simulink model "gm_CustArch_vnl"  (R2020a)
settings: Solver=FixedStepDiscrete  StartTime=0.0  StopTime=7e4  RelTol=1e-3
libraries: simulink x176, hdlsllib x104, hdlmdlgenlib x2, dsparch4 x1
(part 4 of 4)

== system gm_CustArch_vnl/cust_architecture_vnl/output_interpret/Interpret_to_RAM_output/get enabled timings /Subsystem ==
  note: this is the ugliest thing ever--- but it works.. so far so good
  "counter " : Inport
  data_stream_en : Inport  Port=2
  Bit Rotate : hdlsllib/Logic and Bit Operations/Bit Rotate  mode=Rotate Right  N=1
      settings: SourceProductBaseCode=SL
  Bit Rotate1 : hdlsllib/Logic and Bit Operations/Bit Rotate  mode=Rotate Right  N=2
      settings: SourceProductBaseCode=SL
  Bit Rotate2 : hdlsllib/Logic and Bit Operations/Bit Rotate  mode=Rotate Right  N=3
      settings: SourceProductBaseCode=SL
  Bit Rotate3 : hdlsllib/Logic and Bit Operations/Bit Rotate  mode=Rotate Right  N=4
      settings: SourceProductBaseCode=SL
  Bit Rotate4 : hdlsllib/Logic and Bit Operations/Bit Rotate  mode=Rotate Right  N=5
      settings: SourceProductBaseCode=SL
  Bit Rotate5 : hdlsllib/Logic and Bit Operations/Bit Rotate  mode=Rotate Right  N=6
      settings: SourceProductBaseCode=SL
  Bit Rotate6 : hdlsllib/Logic and Bit Operations/Bit Rotate  mode=Rotate Right  N=7
      settings: SourceProductBaseCode=SL
  Bit Slice : hdlsllib/Logic and Bit Operations/Bit Slice  lidx=0  ridx=0
      settings: SourceProductBaseCode=SL
  Compare To Constant : simulink/Logic and Bit Operations/Compare To Constant  relop===  const=0  OutDataTypeStr=boolean
  Compare To Constant1 : simulink/Logic and Bit Operations/Compare To Constant  relop===  const=1  OutDataTypeStr=boolean
  Compare To Constant2 : simulink/Logic and Bit Operations/Compare To Constant  relop===  const=2  OutDataTypeStr=boolean
  Compare To Constant3 : simulink/Logic and Bit Operations/Compare To Constant  relop===  const=3  OutDataTypeStr=boolean
  Compare To Constant4 : simulink/Logic and Bit Operations/Compare To Constant  relop===  const=4  OutDataTypeStr=boolean
  Compare To Constant5 : simulink/Logic and Bit Operations/Compare To Constant  relop===  const=5  OutDataTypeStr=boolean
  Compare To Constant6 : simulink/Logic and Bit Operations/Compare To Constant  relop===  const=6  OutDataTypeStr=boolean
  Compare To Constant7 : simulink/Logic and Bit Operations/Compare To Constant  relop===  const=7  OutDataTypeStr=boolean
  Constant : Constant  Value=0  OutDataTypeStr=uint8  SampleTime=-1
  Switch{,1..7} (8 alike) : Switch  Criteria=u2 > Threshold
  source_device_en : Outport  VectorParamsAs1DForOutWhenUnconnected=off
  source_device : Outport  Port=2  VectorParamsAs1DForOutWhenUnconnected=off
  wires:
  Bit Slice/1 -> source_device_en/1
  Switch/1 -> Bit Slice/1
  data_stream_en/1 -> Bit Rotate6/1, Bit Rotate5/1, Bit Rotate4/1, Bit Rotate3/1, Bit Rotate2/1, Bit Rotate1/1, Bit Rotate/1, Switch/1
  Switch2/1 -> Switch1/3
  Constant/1 -> Switch7/3
  Bit Rotate6/1 -> Switch7/1
  Switch7/1 -> Switch6/3
  Compare To Constant7/1 -> Switch7/2
  Bit Rotate5/1 -> Switch6/1
  Switch6/1 -> Switch5/3
  Compare To Constant6/1 -> Switch6/2
  Switch5/1 -> Switch4/3
  Bit Rotate4/1 -> Switch5/1
  Compare To Constant5/1 -> Switch5/2
  Bit Rotate3/1 -> Switch4/1
  Switch4/1 -> Switch3/3
  Compare To Constant4/1 -> Switch4/2
  Bit Rotate2/1 -> Switch3/1
  Switch3/1 -> Switch2/3
  Compare To Constant3/1 -> Switch3/2
  Bit Rotate1/1 -> Switch2/1
  Compare To Constant2/1 -> Switch2/2
  Switch1/1 -> Switch/3
  "counter "/1 -> source_device/1, Compare To Constant/1, Compare To Constant1/1, Compare To Constant2/1, Compare To Constant3/1, Compare To Constant4/1, Compare To Constant5/1, Compare To Constant6/1, Compare To Constant7/1
  Bit Rotate/1 -> Switch1/1
  Compare To Constant1/1 -> Switch1/2
  Compare To Constant/1 -> Switch/2

== system gm_CustArch_vnl/cust_architecture_vnl/output_interpret/Interpret_to_RAM_output/get enabled timings /Triggered Subsystem ==
  In1 : Inport
  Trigger : TriggerPort  VariantControl=Variant
  Bit Rotate : hdlsllib/Logic and Bit Operations/Bit Rotate  mode=Rotate Right  N=1
      settings: SourceProductBaseCode=SL
  Out1 : Outport  InitialOutput=0  VectorParamsAs1DForOutWhenUnconnected=off
  wires:
  Bit Rotate/1 -> Out1/1
  In1/1 -> Bit Rotate/1

== system gm_CustArch_vnl/cust_architecture/input_interpret_store_retrieve/Interpret_to_RAM_input/interpret data/get_sources/Subsystem ==
  source_device : Inport  OutDataTypeStr=uint8  PortDimensions=1  SampleTime=1
  dev_output : Inport  Port=2  OutDataTypeStr=uint8  PortDimensions=1  SampleTime=1
  Enable : EnablePort  OutDataTypeStr=boolean
  Bit Concat : hdlsllib/Logic and Bit Operations/Bit Concat  numInputs=2
  Bit Slice : hdlsllib/Logic and Bit Operations/Bit Slice  lidx=double(4)  ridx=double(0)
      settings: SourceProductBaseCode=SL
  Bit Slice1 : hdlsllib/Logic and Bit Operations/Bit Slice  lidx=double(2)  ridx=double(0)
      settings: SourceProductBaseCode=SL
  source_channel_0_159 : Outport  InitialOutput=0  VectorParamsAs1DForOutWhenUnconnected=off
  wires:
  Bit Slice1/1 -> Bit Concat/2
  Bit Slice/1 -> Bit Concat/1
  Bit Concat/1 -> source_channel_0_159/1
  dev_output/1 -> Bit Slice/1
  source_device/1 -> Bit Slice1/1

== system gm_CustArch_vnl/cust_architecture/input_interpret_store_retrieve/Interpret_to_RAM_input/interpret data/get_sources/Triggered Subsystem ==
  In1 : Inport  OutDataTypeStr=uint8  PortDimensions=1  SampleTime=1
  Enable : EnablePort  OutDataTypeStr=boolean
  Out1 : Outport  InitialOutput=0  VectorParamsAs1DForOutWhenUnconnected=off
  wires:
  In1/1 -> Out1/1

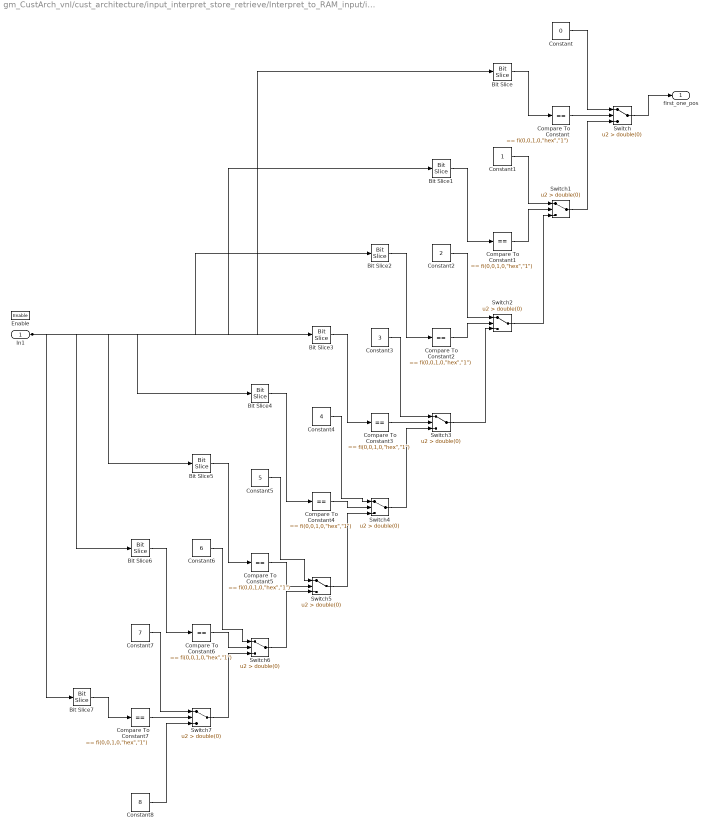
== system gm_CustArch_vnl/cust_architecture/input_interpret_store_retrieve/Interpret_to_RAM_input/interpret data/get_sources/find_first_one_pos ==
  In1 : Inport  OutDataTypeStr=uint8  PortDimensions=1  SampleTime=1
  Enable : EnablePort  OutDataTypeStr=boolean
  Bit Slice : hdlsllib/Logic and Bit Operations/Bit Slice  lidx=double(0)  ridx=double(0)
      settings: SourceProductBaseCode=SL
  Bit Slice1 : hdlsllib/Logic and Bit Operations/Bit Slice  lidx=double(1)  ridx=double(1)
      settings: SourceProductBaseCode=SL
  Bit Slice2 : hdlsllib/Logic and Bit Operations/Bit Slice  lidx=double(2)  ridx=double(2)
      settings: SourceProductBaseCode=SL
  Bit Slice3 : hdlsllib/Logic and Bit Operations/Bit Slice  lidx=double(3)  ridx=double(3)
      settings: SourceProductBaseCode=SL
  Bit Slice4 : hdlsllib/Logic and Bit Operations/Bit Slice  lidx=double(4)  ridx=double(4)
      settings: SourceProductBaseCode=SL
  Bit Slice5 : hdlsllib/Logic and Bit Operations/Bit Slice  lidx=double(5)  ridx=double(5)
      settings: SourceProductBaseCode=SL
  Bit Slice6 : hdlsllib/Logic and Bit Operations/Bit Slice  lidx=double(6)  ridx=double(6)
      settings: SourceProductBaseCode=SL
  Bit Slice7 : hdlsllib/Logic and Bit Operations/Bit Slice  lidx=double(7)  ridx=double(7)
      settings: SourceProductBaseCode=SL
  Compare To Constant{,1..7} (8 alike) : simulink/Logic and Bit Operations/Compare To Constant  relop===  const="fi(0,0,1,0,\"hex\",\"1\")"  OutDataTypeStr=boolean
  Constant : Constant  Value=0  OutDataTypeStr=uint8  SampleTime=1
  Constant1 : Constant  OutDataTypeStr=uint8  SampleTime=1
  Constant2 : Constant  Value=2  OutDataTypeStr=uint8  SampleTime=1
  Constant3 : Constant  Value=3  OutDataTypeStr=uint8  SampleTime=1
  Constant4 : Constant  Value=4  OutDataTypeStr=uint8  SampleTime=1
  Constant5 : Constant  Value=5  OutDataTypeStr=uint8  SampleTime=1
  Constant6 : Constant  Value=6  OutDataTypeStr=uint8  SampleTime=1
  Constant7 : Constant  Value=7  OutDataTypeStr=uint8  SampleTime=1
  Constant8 : Constant  Value=8  OutDataTypeStr=uint8  SampleTime=1
  Switch{,1..7} (8 alike) : Switch  Criteria=u2 > Threshold  Threshold=double(0)  OutDataTypeStr=uint8  SampleTime=1
  first_one_pos : Outport  InitialOutput=0  VectorParamsAs1DForOutWhenUnconnected=off
  wires:
  Switch7/1 -> Switch6/3
  Switch6/1 -> Switch5/3
  Switch5/1 -> Switch4/3
  Switch4/1 -> Switch3/3
  Switch3/1 -> Switch2/3
  Switch2/1 -> Switch1/3
  Switch1/1 -> Switch/3
  Switch/1 -> first_one_pos/1
  Constant8/1 -> Switch7/3
  Constant7/1 -> Switch7/1
  Constant6/1 -> Switch6/1
  Constant5/1 -> Switch5/1
  Constant4/1 -> Switch4/1
  Constant3/1 -> Switch3/1
  Constant2/1 -> Switch2/1
  Constant1/1 -> Switch1/1
  Constant/1 -> Switch/1
  Compare To Constant7/1 -> Switch7/2
  Compare To Constant6/1 -> Switch6/2
  Compare To Constant5/1 -> Switch5/2
  Compare To Constant4/1 -> Switch4/2
  Compare To Constant3/1 -> Switch3/2
  Compare To Constant2/1 -> Switch2/2
  Compare To Constant1/1 -> Switch1/2
  Compare To Constant/1 -> Switch/2
  Bit Slice7/1 -> Compare To Constant7/1
  Bit Slice6/1 -> Compare To Constant6/1
  Bit Slice5/1 -> Compare To Constant5/1
  Bit Slice4/1 -> Compare To Constant4/1
  Bit Slice3/1 -> Compare To Constant3/1
  Bit Slice2/1 -> Compare To Constant2/1
  Bit Slice1/1 -> Compare To Constant1/1
  Bit Slice/1 -> Compare To Constant/1
  In1/1 -> Bit Slice/1, Bit Slice1/1, Bit Slice2/1, Bit Slice3/1, Bit Slice4/1, Bit Slice5/1, Bit Slice6/1, Bit Slice7/1

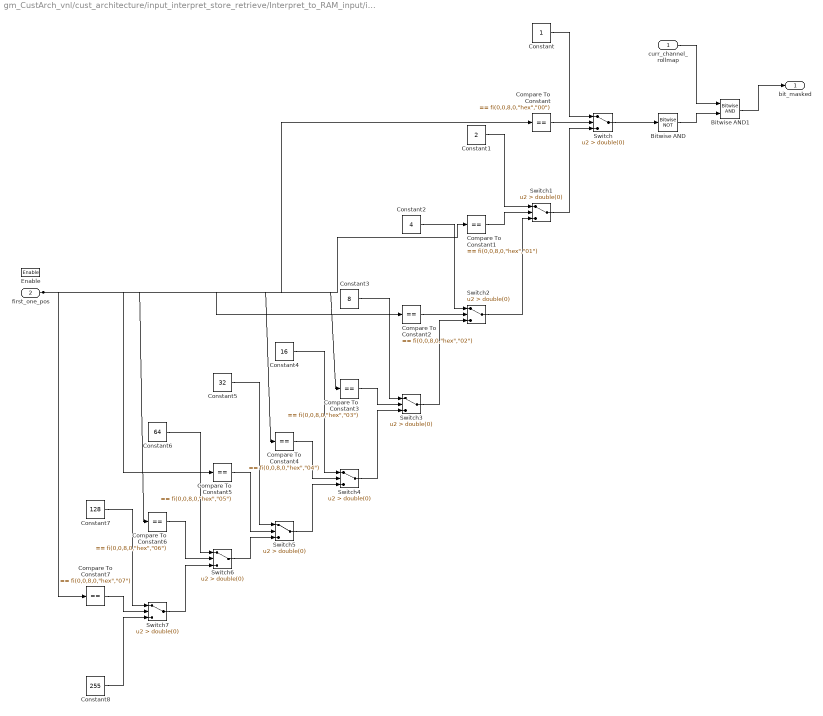
== system gm_CustArch_vnl/cust_architecture/input_interpret_store_retrieve/Interpret_to_RAM_input/interpret data/get_sources/position_to_bitmask ==
  curr_channel_rollmap : Inport  OutDataTypeStr=uint8  PortDimensions=1  SampleTime=1
  first_one_pos : Inport  Port=2  OutDataTypeStr=uint8  PortDimensions=1  SampleTime=1
  Enable : EnablePort  OutDataTypeStr=boolean
  Bitwise AND : simulink/Logic and Bit Operations/Bitwise Operator  logicop=NOT  UseBitMask=off  BitMask=double(0)  BitMaskRealWorld=Real World Value
  Bitwise AND1 : simulink/Logic and Bit Operations/Bitwise Operator  logicop=AND  UseBitMask=off  NumInputPorts=2  BitMask=double(0)  BitMaskRealWorld=Real World Value
  Compare To Constant : simulink/Logic and Bit Operations/Compare To Constant  relop===  const="fi(0,0,8,0,\"hex\",\"00\")"  OutDataTypeStr=boolean
  Compare To Constant1 : simulink/Logic and Bit Operations/Compare To Constant  relop===  const="fi(0,0,8,0,\"hex\",\"01\")"  OutDataTypeStr=boolean
  Compare To Constant2 : simulink/Logic and Bit Operations/Compare To Constant  relop===  const="fi(0,0,8,0,\"hex\",\"02\")"  OutDataTypeStr=boolean
  Compare To Constant3 : simulink/Logic and Bit Operations/Compare To Constant  relop===  const="fi(0,0,8,0,\"hex\",\"03\")"  OutDataTypeStr=boolean
  Compare To Constant4 : simulink/Logic and Bit Operations/Compare To Constant  relop===  const="fi(0,0,8,0,\"hex\",\"04\")"  OutDataTypeStr=boolean
  Compare To Constant5 : simulink/Logic and Bit Operations/Compare To Constant  relop===  const="fi(0,0,8,0,\"hex\",\"05\")"  OutDataTypeStr=boolean
  Compare To Constant6 : simulink/Logic and Bit Operations/Compare To Constant  relop===  const="fi(0,0,8,0,\"hex\",\"06\")"  OutDataTypeStr=boolean
  Compare To Constant7 : simulink/Logic and Bit Operations/Compare To Constant  relop===  const="fi(0,0,8,0,\"hex\",\"07\")"  OutDataTypeStr=boolean
  Constant : Constant  OutDataTypeStr=uint8  SampleTime=1
  Constant1 : Constant  Value=2  OutDataTypeStr=uint8  SampleTime=1
  Constant2 : Constant  Value=4  OutDataTypeStr=uint8  SampleTime=1
  Constant3 : Constant  Value=8  OutDataTypeStr=uint8  SampleTime=1
  Constant4 : Constant  Value=16  OutDataTypeStr=uint8  SampleTime=1
  Constant5 : Constant  Value=32  OutDataTypeStr=uint8  SampleTime=1
  Constant6 : Constant  Value=64  OutDataTypeStr=uint8  SampleTime=1
  Constant7 : Constant  Value=128  OutDataTypeStr=uint8  SampleTime=1
  Constant8 : Constant  Value=255  OutDataTypeStr=uint8  SampleTime=1
  Switch{,1..7} (8 alike) : Switch  Criteria=u2 > Threshold  Threshold=double(0)  OutDataTypeStr=uint8  SampleTime=1
  bit_masked : Outport  InitialOutput=0  VectorParamsAs1DForOutWhenUnconnected=off
  wires:
  Switch7/1 -> Switch6/3
  Switch6/1 -> Switch5/3
  Switch5/1 -> Switch4/3
  Switch4/1 -> Switch3/3
  Switch3/1 -> Switch2/3
  Switch2/1 -> Switch1/3
  Switch1/1 -> Switch/3
  Switch/1 -> Bitwise AND/1
  Constant8/1 -> Switch7/3
  Constant7/1 -> Switch7/1
  Constant6/1 -> Switch6/1
  Constant5/1 -> Switch5/1
  Constant4/1 -> Switch4/1
  Constant3/1 -> Switch3/1
  Constant2/1 -> Switch2/1
  Constant1/1 -> Switch1/1
  Constant/1 -> Switch/1
  Compare To Constant7/1 -> Switch7/2
  Compare To Constant6/1 -> Switch6/2
  Compare To Constant5/1 -> Switch5/2
  Compare To Constant4/1 -> Switch4/2
  Compare To Constant3/1 -> Switch3/2
  Compare To Constant2/1 -> Switch2/2
  Compare To Constant1/1 -> Switch1/2
  Compare To Constant/1 -> Switch/2
  Bitwise AND1/1 -> bit_masked/1
  Bitwise AND/1 -> Bitwise AND1/2
  first_one_pos/1 -> Compare To Constant/1, Compare To Constant1/1, Compare To Constant2/1, Compare To Constant3/1, Compare To Constant4/1, Compare To Constant5/1, Compare To Constant6/1, Compare To Constant7/1
  curr_channel_rollmap/1 -> Bitwise AND1/1

== system gm_CustArch_vnl/cust_architecture/process_and_retrieve/80-120Hz IIR/controlss_temp/Filter/delay_process_section10_tap0 ==
  in0 : Inport  OutDataTypeStr=fixdt(1, 16, 15)  SampleTime=1
  Trigger_emulated : EnablePort  OutDataTypeStr=boolean
  delay_process_section10_tap0 : Delay  DelayLength=double(1)
  out0 : Outport  OutDataTypeStr=fixdt(1, 16, 15)  InitialOutput=0
  wires:
  in0/1 -> delay_process_section10_tap0/1
  delay_process_section10_tap0/1 -> out0/1

== system gm_CustArch_vnl/cust_architecture/process_and_retrieve/80-120Hz IIR/controlss_temp/Filter/delay_process_section10_tap1 ==
  in0 : Inport  OutDataTypeStr=fixdt(1, 16, 15)  SampleTime=1
  Trigger_emulated : EnablePort  OutDataTypeStr=boolean
  delay_process_section10_tap1 : Delay  DelayLength=double(1)
  out0 : Outport  OutDataTypeStr=fixdt(1, 16, 15)  InitialOutput=0
  wires:
  in0/1 -> delay_process_section10_tap1/1
  delay_process_section10_tap1/1 -> out0/1

== system gm_CustArch_vnl/cust_architecture/process_and_retrieve/80-120Hz IIR/controlss_temp/Filter/delay_process_section11_tap0 ==
  in0 : Inport  OutDataTypeStr=fixdt(1, 16, 15)  SampleTime=1
  Trigger_emulated : EnablePort  OutDataTypeStr=boolean
  delay_process_section11_tap0 : Delay  DelayLength=double(1)
  out0 : Outport  OutDataTypeStr=fixdt(1, 16, 15)  InitialOutput=0
  wires:
  in0/1 -> delay_process_section11_tap0/1
  delay_process_section11_tap0/1 -> out0/1

== system gm_CustArch_vnl/cust_architecture/process_and_retrieve/80-120Hz IIR/controlss_temp/Filter/delay_process_section11_tap1 ==
  in0 : Inport  OutDataTypeStr=fixdt(1, 16, 15)  SampleTime=1
  Trigger_emulated : EnablePort  OutDataTypeStr=boolean
  delay_process_section11_tap1 : Delay  DelayLength=double(1)
  out0 : Outport  OutDataTypeStr=fixdt(1, 16, 15)  InitialOutput=0
  wires:
  in0/1 -> delay_process_section11_tap1/1
  delay_process_section11_tap1/1 -> out0/1

== system gm_CustArch_vnl/cust_architecture/process_and_retrieve/80-120Hz IIR/controlss_temp/Filter/delay_process_section12_tap0 ==
  in0 : Inport  OutDataTypeStr=fixdt(1, 16, 15)  SampleTime=1
  Trigger_emulated : EnablePort  OutDataTypeStr=boolean
  delay_process_section12_tap0 : Delay  DelayLength=double(1)
  out0 : Outport  OutDataTypeStr=fixdt(1, 16, 15)  InitialOutput=0
  wires:
  in0/1 -> delay_process_section12_tap0/1
  delay_process_section12_tap0/1 -> out0/1

== system gm_CustArch_vnl/cust_architecture/process_and_retrieve/80-120Hz IIR/controlss_temp/Filter/delay_process_section12_tap1 ==
  in0 : Inport  OutDataTypeStr=fixdt(1, 16, 15)  SampleTime=1
  Trigger_emulated : EnablePort  OutDataTypeStr=boolean
  delay_process_section12_tap1 : Delay  DelayLength=double(1)
  out0 : Outport  OutDataTypeStr=fixdt(1, 16, 15)  InitialOutput=0
  wires:
  in0/1 -> delay_process_section12_tap1/1
  delay_process_section12_tap1/1 -> out0/1

== system gm_CustArch_vnl/cust_architecture/process_and_retrieve/80-120Hz IIR/controlss_temp/Filter/delay_process_section13_tap0 ==
  in0 : Inport  OutDataTypeStr=fixdt(1, 16, 15)  SampleTime=1
  Trigger_emulated : EnablePort  OutDataTypeStr=boolean
  delay_process_section13_tap0 : Delay  DelayLength=double(1)
  out0 : Outport  OutDataTypeStr=fixdt(1, 16, 15)  InitialOutput=0
  wires:
  in0/1 -> delay_process_section13_tap0/1
  delay_process_section13_tap0/1 -> out0/1

== system gm_CustArch_vnl/cust_architecture/process_and_retrieve/80-120Hz IIR/controlss_temp/Filter/delay_process_section13_tap1 ==
  in0 : Inport  OutDataTypeStr=fixdt(1, 16, 15)  SampleTime=1
  Trigger_emulated : EnablePort  OutDataTypeStr=boolean
  delay_process_section13_tap1 : Delay  DelayLength=double(1)
  out0 : Outport  OutDataTypeStr=fixdt(1, 16, 15)  InitialOutput=0
  wires:
  in0/1 -> delay_process_section13_tap1/1
  delay_process_section13_tap1/1 -> out0/1

== system gm_CustArch_vnl/cust_architecture/process_and_retrieve/80-120Hz IIR/controlss_temp/Filter/delay_process_section14_tap0 ==
  in0 : Inport  OutDataTypeStr=fixdt(1, 16, 15)  SampleTime=1
  Trigger_emulated : EnablePort  OutDataTypeStr=boolean
  delay_process_section14_tap0 : Delay  DelayLength=double(1)
  out0 : Outport  OutDataTypeStr=fixdt(1, 16, 15)  InitialOutput=0
  wires:
  in0/1 -> delay_process_section14_tap0/1
  delay_process_section14_tap0/1 -> out0/1

== system gm_CustArch_vnl/cust_architecture/process_and_retrieve/80-120Hz IIR/controlss_temp/Filter/delay_process_section14_tap1 ==
  in0 : Inport  OutDataTypeStr=fixdt(1, 16, 15)  SampleTime=1
  Trigger_emulated : EnablePort  OutDataTypeStr=boolean
  delay_process_section14_tap1 : Delay  DelayLength=double(1)
  out0 : Outport  OutDataTypeStr=fixdt(1, 16, 15)  InitialOutput=0
  wires:
  in0/1 -> delay_process_section14_tap1/1
  delay_process_section14_tap1/1 -> out0/1

== system gm_CustArch_vnl/cust_architecture/process_and_retrieve/80-120Hz IIR/controlss_temp/Filter/delay_process_section15_tap0 ==
  in0 : Inport  OutDataTypeStr=fixdt(1, 16, 15)  SampleTime=1
  Trigger_emulated : EnablePort  OutDataTypeStr=boolean
  delay_process_section15_tap0 : Delay  DelayLength=double(1)
  out0 : Outport  OutDataTypeStr=fixdt(1, 16, 15)  InitialOutput=0
  wires:
  in0/1 -> delay_process_section15_tap0/1
  delay_process_section15_tap0/1 -> out0/1

== system gm_CustArch_vnl/cust_architecture/process_and_retrieve/80-120Hz IIR/controlss_temp/Filter/delay_process_section15_tap1 ==
  in0 : Inport  OutDataTypeStr=fixdt(1, 16, 15)  SampleTime=1
  Trigger_emulated : EnablePort  OutDataTypeStr=boolean
  delay_process_section15_tap1 : Delay  DelayLength=double(1)
  out0 : Outport  OutDataTypeStr=fixdt(1, 16, 15)  InitialOutput=0
  wires:
  in0/1 -> delay_process_section15_tap1/1
  delay_process_section15_tap1/1 -> out0/1

== system gm_CustArch_vnl/cust_architecture/process_and_retrieve/80-120Hz IIR/controlss_temp/Filter/delay_process_section16_tap0 ==
  in0 : Inport  OutDataTypeStr=fixdt(1, 16, 15)  SampleTime=1
  Trigger_emulated : EnablePort  OutDataTypeStr=boolean
  delay_process_section16_tap0 : Delay  DelayLength=double(1)
  out0 : Outport  OutDataTypeStr=fixdt(1, 16, 15)  InitialOutput=0
  wires:
  in0/1 -> delay_process_section16_tap0/1
  delay_process_section16_tap0/1 -> out0/1

== system gm_CustArch_vnl/cust_architecture/process_and_retrieve/80-120Hz IIR/controlss_temp/Filter/delay_process_section16_tap1 ==
  in0 : Inport  OutDataTypeStr=fixdt(1, 16, 15)  SampleTime=1
  Trigger_emulated : EnablePort  OutDataTypeStr=boolean
  delay_process_section16_tap1 : Delay  DelayLength=double(1)
  out0 : Outport  OutDataTypeStr=fixdt(1, 16, 15)  InitialOutput=0
  wires:
  in0/1 -> delay_process_section16_tap1/1
  delay_process_section16_tap1/1 -> out0/1

== system gm_CustArch_vnl/cust_architecture/process_and_retrieve/80-120Hz IIR/controlss_temp/Filter/delay_process_section17_tap0 ==
  in0 : Inport  OutDataTypeStr=fixdt(1, 16, 15)  SampleTime=1
  Trigger_emulated : EnablePort  OutDataTypeStr=boolean
  delay_process_section17_tap0 : Delay  DelayLength=double(1)
  out0 : Outport  OutDataTypeStr=fixdt(1, 16, 15)  InitialOutput=0
  wires:
  in0/1 -> delay_process_section17_tap0/1
  delay_process_section17_tap0/1 -> out0/1

== system gm_CustArch_vnl/cust_architecture/process_and_retrieve/80-120Hz IIR/controlss_temp/Filter/delay_process_section17_tap1 ==
  in0 : Inport  OutDataTypeStr=fixdt(1, 16, 15)  SampleTime=1
  Trigger_emulated : EnablePort  OutDataTypeStr=boolean
  delay_process_section17_tap1 : Delay  DelayLength=double(1)
  out0 : Outport  OutDataTypeStr=fixdt(1, 16, 15)  InitialOutput=0
  wires:
  in0/1 -> delay_process_section17_tap1/1
  delay_process_section17_tap1/1 -> out0/1

== system gm_CustArch_vnl/cust_architecture/process_and_retrieve/80-120Hz IIR/controlss_temp/Filter/delay_process_section18_tap0 ==
  in0 : Inport  OutDataTypeStr=fixdt(1, 16, 15)  SampleTime=1
  Trigger_emulated : EnablePort  OutDataTypeStr=boolean
  delay_process_section18_tap0 : Delay  DelayLength=double(1)
  out0 : Outport  OutDataTypeStr=fixdt(1, 16, 15)  InitialOutput=0
  wires:
  in0/1 -> delay_process_section18_tap0/1
  delay_process_section18_tap0/1 -> out0/1

== system gm_CustArch_vnl/cust_architecture/process_and_retrieve/80-120Hz IIR/controlss_temp/Filter/delay_process_section18_tap1 ==
  in0 : Inport  OutDataTypeStr=fixdt(1, 16, 15)  SampleTime=1
  Trigger_emulated : EnablePort  OutDataTypeStr=boolean
  delay_process_section18_tap1 : Delay  DelayLength=double(1)
  out0 : Outport  OutDataTypeStr=fixdt(1, 16, 15)  InitialOutput=0
  wires:
  in0/1 -> delay_process_section18_tap1/1
  delay_process_section18_tap1/1 -> out0/1

== system gm_CustArch_vnl/cust_architecture/process_and_retrieve/80-120Hz IIR/controlss_temp/Filter/delay_process_section1_tap0 ==
  in0 : Inport  OutDataTypeStr=fixdt(1, 16, 15)  SampleTime=1
  Trigger_emulated : EnablePort  OutDataTypeStr=boolean
  delay_process_section1_tap0 : Delay  DelayLength=double(1)
  out0 : Outport  OutDataTypeStr=fixdt(1, 16, 15)  InitialOutput=0
  wires:
  in0/1 -> delay_process_section1_tap0/1
  delay_process_section1_tap0/1 -> out0/1

== system gm_CustArch_vnl/cust_architecture/process_and_retrieve/80-120Hz IIR/controlss_temp/Filter/delay_process_section1_tap1 ==
  in0 : Inport  OutDataTypeStr=fixdt(1, 16, 15)  SampleTime=1
  Trigger_emulated : EnablePort  OutDataTypeStr=boolean
  delay_process_section1_tap1 : Delay  DelayLength=double(1)
  out0 : Outport  OutDataTypeStr=fixdt(1, 16, 15)  InitialOutput=0
  wires:
  in0/1 -> delay_process_section1_tap1/1
  delay_process_section1_tap1/1 -> out0/1

== system gm_CustArch_vnl/cust_architecture/process_and_retrieve/80-120Hz IIR/controlss_temp/Filter/delay_process_section2_tap0 ==
  in0 : Inport  OutDataTypeStr=fixdt(1, 16, 15)  SampleTime=1
  Trigger_emulated : EnablePort  OutDataTypeStr=boolean
  delay_process_section2_tap0 : Delay  DelayLength=double(1)
  out0 : Outport  OutDataTypeStr=fixdt(1, 16, 15)  InitialOutput=0
  wires:
  in0/1 -> delay_process_section2_tap0/1
  delay_process_section2_tap0/1 -> out0/1

== system gm_CustArch_vnl/cust_architecture/process_and_retrieve/80-120Hz IIR/controlss_temp/Filter/delay_process_section2_tap1 ==
  in0 : Inport  OutDataTypeStr=fixdt(1, 16, 15)  SampleTime=1
  Trigger_emulated : EnablePort  OutDataTypeStr=boolean
  delay_process_section2_tap1 : Delay  DelayLength=double(1)
  out0 : Outport  OutDataTypeStr=fixdt(1, 16, 15)  InitialOutput=0
  wires:
  in0/1 -> delay_process_section2_tap1/1
  delay_process_section2_tap1/1 -> out0/1

== system gm_CustArch_vnl/cust_architecture/process_and_retrieve/80-120Hz IIR/controlss_temp/Filter/delay_process_section3_tap0 ==
  in0 : Inport  OutDataTypeStr=fixdt(1, 16, 15)  SampleTime=1
  Trigger_emulated : EnablePort  OutDataTypeStr=boolean
  delay_process_section3_tap0 : Delay  DelayLength=double(1)
  out0 : Outport  OutDataTypeStr=fixdt(1, 16, 15)  InitialOutput=0
  wires:
  in0/1 -> delay_process_section3_tap0/1
  delay_process_section3_tap0/1 -> out0/1

== system gm_CustArch_vnl/cust_architecture/process_and_retrieve/80-120Hz IIR/controlss_temp/Filter/delay_process_section3_tap1 ==
  in0 : Inport  OutDataTypeStr=fixdt(1, 16, 15)  SampleTime=1
  Trigger_emulated : EnablePort  OutDataTypeStr=boolean
  delay_process_section3_tap1 : Delay  DelayLength=double(1)
  out0 : Outport  OutDataTypeStr=fixdt(1, 16, 15)  InitialOutput=0
  wires:
  in0/1 -> delay_process_section3_tap1/1
  delay_process_section3_tap1/1 -> out0/1

== system gm_CustArch_vnl/cust_architecture/process_and_retrieve/80-120Hz IIR/controlss_temp/Filter/delay_process_section4_tap0 ==
  in0 : Inport  OutDataTypeStr=fixdt(1, 16, 15)  SampleTime=1
  Trigger_emulated : EnablePort  OutDataTypeStr=boolean
  delay_process_section4_tap0 : Delay  DelayLength=double(1)
  out0 : Outport  OutDataTypeStr=fixdt(1, 16, 15)  InitialOutput=0
  wires:
  in0/1 -> delay_process_section4_tap0/1
  delay_process_section4_tap0/1 -> out0/1

== system gm_CustArch_vnl/cust_architecture/process_and_retrieve/80-120Hz IIR/controlss_temp/Filter/delay_process_section4_tap1 ==
  in0 : Inport  OutDataTypeStr=fixdt(1, 16, 15)  SampleTime=1
  Trigger_emulated : EnablePort  OutDataTypeStr=boolean
  delay_process_section4_tap1 : Delay  DelayLength=double(1)
  out0 : Outport  OutDataTypeStr=fixdt(1, 16, 15)  InitialOutput=0
  wires:
  in0/1 -> delay_process_section4_tap1/1
  delay_process_section4_tap1/1 -> out0/1

== system gm_CustArch_vnl/cust_architecture/process_and_retrieve/80-120Hz IIR/controlss_temp/Filter/delay_process_section5_tap0 ==
  in0 : Inport  OutDataTypeStr=fixdt(1, 16, 15)  SampleTime=1
  Trigger_emulated : EnablePort  OutDataTypeStr=boolean
  delay_process_section5_tap0 : Delay  DelayLength=double(1)
  out0 : Outport  OutDataTypeStr=fixdt(1, 16, 15)  InitialOutput=0
  wires:
  in0/1 -> delay_process_section5_tap0/1
  delay_process_section5_tap0/1 -> out0/1

== system gm_CustArch_vnl/cust_architecture/process_and_retrieve/80-120Hz IIR/controlss_temp/Filter/delay_process_section5_tap1 ==
  in0 : Inport  OutDataTypeStr=fixdt(1, 16, 15)  SampleTime=1
  Trigger_emulated : EnablePort  OutDataTypeStr=boolean
  delay_process_section5_tap1 : Delay  DelayLength=double(1)
  out0 : Outport  OutDataTypeStr=fixdt(1, 16, 15)  InitialOutput=0
  wires:
  in0/1 -> delay_process_section5_tap1/1
  delay_process_section5_tap1/1 -> out0/1

== system gm_CustArch_vnl/cust_architecture/process_and_retrieve/80-120Hz IIR/controlss_temp/Filter/delay_process_section6_tap0 ==
  in0 : Inport  OutDataTypeStr=fixdt(1, 16, 15)  SampleTime=1
  Trigger_emulated : EnablePort  OutDataTypeStr=boolean
  delay_process_section6_tap0 : Delay  DelayLength=double(1)
  out0 : Outport  OutDataTypeStr=fixdt(1, 16, 15)  InitialOutput=0
  wires:
  in0/1 -> delay_process_section6_tap0/1
  delay_process_section6_tap0/1 -> out0/1

== system gm_CustArch_vnl/cust_architecture/process_and_retrieve/80-120Hz IIR/controlss_temp/Filter/delay_process_section6_tap1 ==
  in0 : Inport  OutDataTypeStr=fixdt(1, 16, 15)  SampleTime=1
  Trigger_emulated : EnablePort  OutDataTypeStr=boolean
  delay_process_section6_tap1 : Delay  DelayLength=double(1)
  out0 : Outport  OutDataTypeStr=fixdt(1, 16, 15)  InitialOutput=0
  wires:
  in0/1 -> delay_process_section6_tap1/1
  delay_process_section6_tap1/1 -> out0/1

== system gm_CustArch_vnl/cust_architecture/process_and_retrieve/80-120Hz IIR/controlss_temp/Filter/delay_process_section7_tap0 ==
  in0 : Inport  OutDataTypeStr=fixdt(1, 16, 15)  SampleTime=1
  Trigger_emulated : EnablePort  OutDataTypeStr=boolean
  delay_process_section7_tap0 : Delay  DelayLength=double(1)
  out0 : Outport  OutDataTypeStr=fixdt(1, 16, 15)  InitialOutput=0
  wires:
  in0/1 -> delay_process_section7_tap0/1
  delay_process_section7_tap0/1 -> out0/1

== system gm_CustArch_vnl/cust_architecture/process_and_retrieve/80-120Hz IIR/controlss_temp/Filter/delay_process_section7_tap1 ==
  in0 : Inport  OutDataTypeStr=fixdt(1, 16, 15)  SampleTime=1
  Trigger_emulated : EnablePort  OutDataTypeStr=boolean
  delay_process_section7_tap1 : Delay  DelayLength=double(1)
  out0 : Outport  OutDataTypeStr=fixdt(1, 16, 15)  InitialOutput=0
  wires:
  in0/1 -> delay_process_section7_tap1/1
  delay_process_section7_tap1/1 -> out0/1

== system gm_CustArch_vnl/cust_architecture/process_and_retrieve/80-120Hz IIR/controlss_temp/Filter/delay_process_section8_tap0 ==
  in0 : Inport  OutDataTypeStr=fixdt(1, 16, 15)  SampleTime=1
  Trigger_emulated : EnablePort  OutDataTypeStr=boolean
  delay_process_section8_tap0 : Delay  DelayLength=double(1)
  out0 : Outport  OutDataTypeStr=fixdt(1, 16, 15)  InitialOutput=0
  wires:
  in0/1 -> delay_process_section8_tap0/1
  delay_process_section8_tap0/1 -> out0/1

== system gm_CustArch_vnl/cust_architecture/process_and_retrieve/80-120Hz IIR/controlss_temp/Filter/delay_process_section8_tap1 ==
  in0 : Inport  OutDataTypeStr=fixdt(1, 16, 15)  SampleTime=1
  Trigger_emulated : EnablePort  OutDataTypeStr=boolean
  delay_process_section8_tap1 : Delay  DelayLength=double(1)
  out0 : Outport  OutDataTypeStr=fixdt(1, 16, 15)  InitialOutput=0
  wires:
  in0/1 -> delay_process_section8_tap1/1
  delay_process_section8_tap1/1 -> out0/1

== system gm_CustArch_vnl/cust_architecture/process_and_retrieve/80-120Hz IIR/controlss_temp/Filter/delay_process_section9_tap0 ==
  in0 : Inport  OutDataTypeStr=fixdt(1, 16, 15)  SampleTime=1
  Trigger_emulated : EnablePort  OutDataTypeStr=boolean
  delay_process_section9_tap0 : Delay  DelayLength=double(1)
  out0 : Outport  OutDataTypeStr=fixdt(1, 16, 15)  InitialOutput=0
  wires:
  in0/1 -> delay_process_section9_tap0/1
  delay_process_section9_tap0/1 -> out0/1

== system gm_CustArch_vnl/cust_architecture/process_and_retrieve/80-120Hz IIR/controlss_temp/Filter/delay_process_section9_tap1 ==
  in0 : Inport  OutDataTypeStr=fixdt(1, 16, 15)  SampleTime=1
  Trigger_emulated : EnablePort  OutDataTypeStr=boolean
  delay_process_section9_tap1 : Delay  DelayLength=double(1)
  out0 : Outport  OutDataTypeStr=fixdt(1, 16, 15)  InitialOutput=0
  wires:
  in0/1 -> delay_process_section9_tap1/1
  delay_process_section9_tap1/1 -> out0/1

== system gm_CustArch_vnl/cust_architecture_vnl/input_interpret_store_retrieve/Interpret_to_RAM_input/interpret data/get_sources/Subsystem ==
  source_device : Inport
  dev_output : Inport  Port=2
  Enable : EnablePort
  Bit Concat : hdlsllib/Logic and Bit Operations/Bit Concat  numInputs=2
  Bit Slice : hdlsllib/Logic and Bit Operations/Bit Slice  lidx=4  ridx=0
      settings: SourceProductBaseCode=SL
  Bit Slice1 : hdlsllib/Logic and Bit Operations/Bit Slice  lidx=2  ridx=0
      settings: SourceProductBaseCode=SL
  source_channel_0_159 : Outport  InitialOutput=0  VectorParamsAs1DForOutWhenUnconnected=off
  wires:
  dev_output/1 -> Bit Slice/1
  Bit Concat/1 -> source_channel_0_159/1  "source_channel_0_159"
  Bit Slice1/1 -> Bit Concat/2
  Bit Slice/1 -> Bit Concat/1
  source_device/1 -> Bit Slice1/1

== system gm_CustArch_vnl/cust_architecture_vnl/input_interpret_store_retrieve/Interpret_to_RAM_input/interpret data/get_sources/Triggered Subsystem ==
  In1 : Inport
  Enable : EnablePort
  Out1 : Outport  InitialOutput=0  VectorParamsAs1DForOutWhenUnconnected=off
  wires:
  In1/1 -> Out1/1

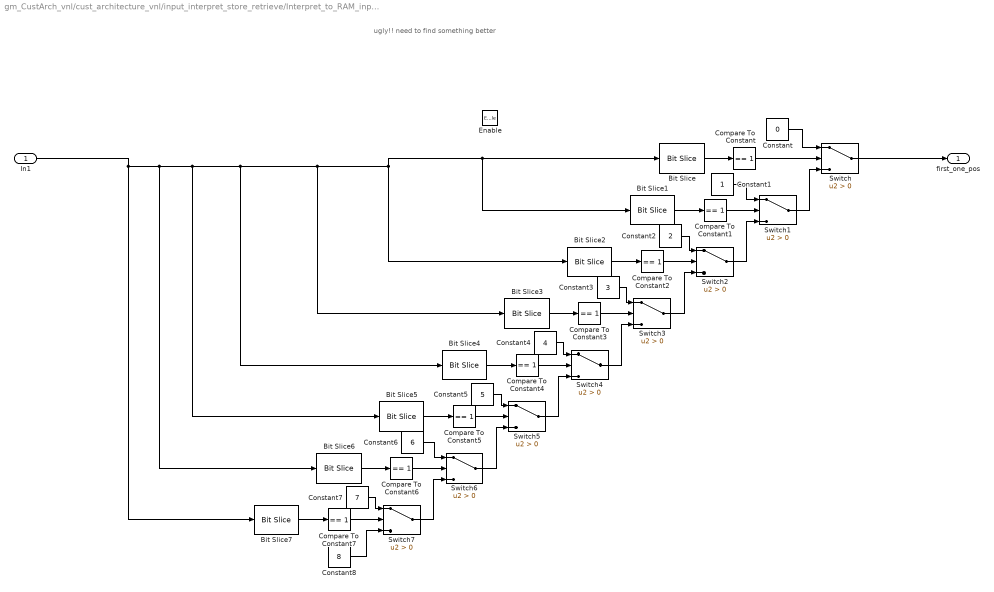
== system gm_CustArch_vnl/cust_architecture_vnl/input_interpret_store_retrieve/Interpret_to_RAM_input/interpret data/get_sources/find_first_one_pos ==
  note: ugly!! need to find something better
  In1 : Inport
  Enable : EnablePort
  Bit Slice : hdlsllib/Logic and Bit Operations/Bit Slice  lidx=0  ridx=0
      settings: SourceProductBaseCode=SL
  Bit Slice1 : hdlsllib/Logic and Bit Operations/Bit Slice  lidx=1  ridx=1
      settings: SourceProductBaseCode=SL
  Bit Slice2 : hdlsllib/Logic and Bit Operations/Bit Slice  lidx=2  ridx=2
      settings: SourceProductBaseCode=SL
  Bit Slice3 : hdlsllib/Logic and Bit Operations/Bit Slice  lidx=3  ridx=3
      settings: SourceProductBaseCode=SL
  Bit Slice4 : hdlsllib/Logic and Bit Operations/Bit Slice  lidx=4  ridx=4
      settings: SourceProductBaseCode=SL
  Bit Slice5 : hdlsllib/Logic and Bit Operations/Bit Slice  lidx=5  ridx=5
      settings: SourceProductBaseCode=SL
  Bit Slice6 : hdlsllib/Logic and Bit Operations/Bit Slice  lidx=6  ridx=6
      settings: SourceProductBaseCode=SL
  Bit Slice7 : hdlsllib/Logic and Bit Operations/Bit Slice  lidx=7  ridx=7
      settings: SourceProductBaseCode=SL
  Compare To Constant{,1..7} (8 alike) : simulink/Logic and Bit Operations/Compare To Constant  relop===  const=1  OutDataTypeStr=boolean
  Constant : Constant  Value=0  OutDataTypeStr=uint8  SampleTime=-1
  Constant1 : Constant  OutDataTypeStr=uint8  SampleTime=-1
  Constant2 : Constant  Value=2  OutDataTypeStr=uint8  SampleTime=-1
  Constant3 : Constant  Value=3  OutDataTypeStr=uint8  SampleTime=-1
  Constant4 : Constant  Value=4  OutDataTypeStr=uint8  SampleTime=-1
  Constant5 : Constant  Value=5  OutDataTypeStr=uint8  SampleTime=-1
  Constant6 : Constant  Value=6  OutDataTypeStr=uint8  SampleTime=-1
  Constant7 : Constant  Value=7  OutDataTypeStr=uint8  SampleTime=-1
  Constant8 : Constant  Value=8  OutDataTypeStr=uint8  SampleTime=-1
  Switch{,1..7} (8 alike) : Switch  Criteria=u2 > Threshold
  first_one_pos : Outport  InitialOutput=0  VectorParamsAs1DForOutWhenUnconnected=off
  wires:
  In1/1 -> Bit Slice/1, Bit Slice1/1, Bit Slice2/1, Bit Slice3/1, Bit Slice4/1, Bit Slice5/1, Bit Slice6/1, Bit Slice7/1
  Constant8/1 -> Switch7/3
  Constant7/1 -> Switch7/1
  Constant6/1 -> Switch6/1
  Constant5/1 -> Switch5/1
  Constant4/1 -> Switch4/1
  Constant3/1 -> Switch3/1
  Constant2/1 -> Switch2/1
  Constant1/1 -> Switch1/1
  Constant/1 -> Switch/1
  Bit Slice7/1 -> Compare To Constant7/1
  Compare To Constant7/1 -> Switch7/2
  Switch7/1 -> Switch6/3
  Switch6/1 -> Switch5/3
  Compare To Constant6/1 -> Switch6/2
  Bit Slice6/1 -> Compare To Constant6/1
  Switch5/1 -> Switch4/3
  Compare To Constant5/1 -> Switch5/2
  Bit Slice5/1 -> Compare To Constant5/1
  Compare To Constant4/1 -> Switch4/2
  Bit Slice4/1 -> Compare To Constant4/1
  Switch4/1 -> Switch3/3
  Switch3/1 -> Switch2/3
  Compare To Constant3/1 -> Switch3/2
  Bit Slice3/1 -> Compare To Constant3/1
  Switch2/1 -> Switch1/3
  Compare To Constant2/1 -> Switch2/2
  Bit Slice2/1 -> Compare To Constant2/1
  Compare To Constant1/1 -> Switch1/2
  Switch1/1 -> Switch/3
  Bit Slice1/1 -> Compare To Constant1/1
  Switch/1 -> first_one_pos/1
  Bit Slice/1 -> Compare To Constant/1
  Compare To Constant/1 -> Switch/2

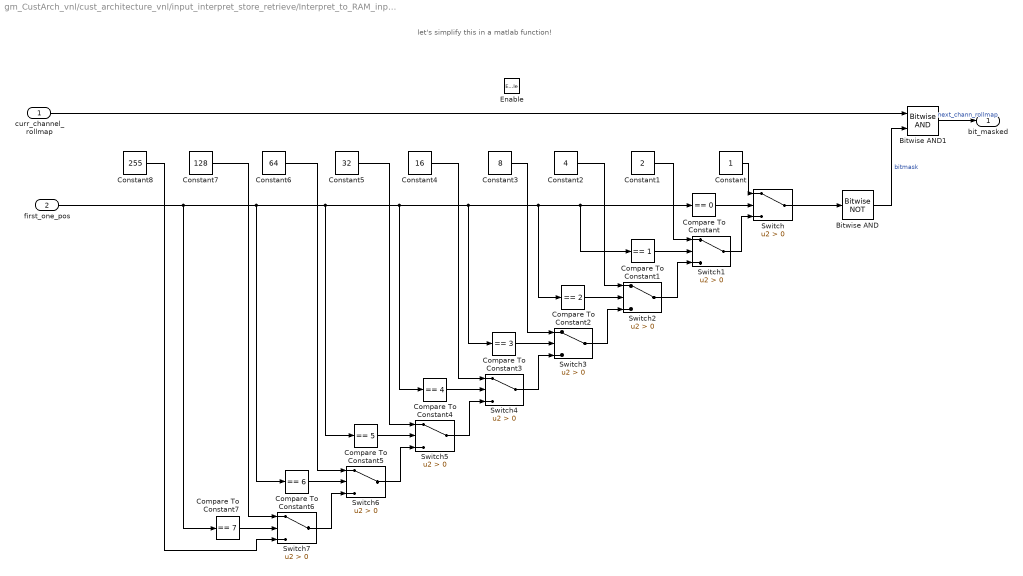
== system gm_CustArch_vnl/cust_architecture_vnl/input_interpret_store_retrieve/Interpret_to_RAM_input/interpret data/get_sources/position_to_bitmask ==
  note: let's simplify this in a matlab function!
  curr_channel_rollmap : Inport
  first_one_pos : Inport  Port=2
  Enable : EnablePort
  Bitwise AND : simulink/Logic and Bit Operations/Bitwise Operator  logicop=NOT  UseBitMask=off  BitMask=bin2dec('11011001')  BitMaskRealWorld=Stored Integer
  Bitwise AND1 : simulink/Logic and Bit Operations/Bitwise Operator  logicop=AND  UseBitMask=off  NumInputPorts=2  BitMask=bin2dec('11011001')  BitMaskRealWorld=Stored Integer
  Compare To Constant : simulink/Logic and Bit Operations/Compare To Constant  relop===  const=0  OutDataTypeStr=boolean
  Compare To Constant1 : simulink/Logic and Bit Operations/Compare To Constant  relop===  const=1  OutDataTypeStr=boolean
  Compare To Constant2 : simulink/Logic and Bit Operations/Compare To Constant  relop===  const=2  OutDataTypeStr=boolean
  Compare To Constant3 : simulink/Logic and Bit Operations/Compare To Constant  relop===  const=3  OutDataTypeStr=boolean
  Compare To Constant4 : simulink/Logic and Bit Operations/Compare To Constant  relop===  const=4  OutDataTypeStr=boolean
  Compare To Constant5 : simulink/Logic and Bit Operations/Compare To Constant  relop===  const=5  OutDataTypeStr=boolean
  Compare To Constant6 : simulink/Logic and Bit Operations/Compare To Constant  relop===  const=6  OutDataTypeStr=boolean
  Compare To Constant7 : simulink/Logic and Bit Operations/Compare To Constant  relop===  const=7  OutDataTypeStr=boolean
  Constant : Constant  OutDataTypeStr=uint8  SampleTime=-1
  Constant1 : Constant  Value=2  OutDataTypeStr=uint8  SampleTime=-1
  Constant2 : Constant  Value=4  OutDataTypeStr=uint8  SampleTime=-1
  Constant3 : Constant  Value=8  OutDataTypeStr=uint8  SampleTime=-1
  Constant4 : Constant  Value=16  OutDataTypeStr=uint8  SampleTime=-1
  Constant5 : Constant  Value=32  OutDataTypeStr=uint8  SampleTime=-1
  Constant6 : Constant  Value=64  OutDataTypeStr=uint8  SampleTime=-1
  Constant7 : Constant  Value=128  OutDataTypeStr=uint8  SampleTime=-1
  Constant8 : Constant  Value=255  OutDataTypeStr=uint8  SampleTime=-1
  Switch{,1..7} (8 alike) : Switch  Criteria=u2 > Threshold
  bit_masked : Outport  InitialOutput=0  VectorParamsAs1DForOutWhenUnconnected=off
  wires:
  Bitwise AND1/1 -> bit_masked/1  "next_chann_rollmap"
  curr_channel_rollmap/1 -> Bitwise AND1/1
  Bitwise AND/1 -> Bitwise AND1/2  "bitmask"
  Constant8/1 -> Switch7/3
  Constant7/1 -> Switch7/1
  first_one_pos/1 -> Compare To Constant/1, Compare To Constant1/1, Compare To Constant2/1, Compare To Constant3/1, Compare To Constant4/1, Compare To Constant5/1, Compare To Constant6/1, Compare To Constant7/1
  Compare To Constant7/1 -> Switch7/2
  Switch7/1 -> Switch6/3
  Constant6/1 -> Switch6/1
  Compare To Constant6/1 -> Switch6/2
  Switch6/1 -> Switch5/3
  Constant5/1 -> Switch5/1
  Switch5/1 -> Switch4/3
  Compare To Constant5/1 -> Switch5/2
  Constant4/1 -> Switch4/1
  Switch4/1 -> Switch3/3
  Compare To Constant4/1 -> Switch4/2
  Constant3/1 -> Switch3/1
  Compare To Constant3/1 -> Switch3/2
  Switch3/1 -> Switch2/3
  Constant2/1 -> Switch2/1
  Switch2/1 -> Switch1/3
  Compare To Constant2/1 -> Switch2/2
  Constant1/1 -> Switch1/1
  Switch1/1 -> Switch/3
  Compare To Constant1/1 -> Switch1/2
  Switch/1 -> Bitwise AND/1
  Constant/1 -> Switch/1
  Compare To Constant/1 -> Switch/2

== stateflow chart gm_CustArch_vnl/cust_architecture/output_interpret/OutputStateMachine/OutputStateMachine ==
  settings: sampleTime=1/1e6  stateMachineType=MOORE_MACHINE  initializeOutput=1
  state idle_state
    OutputState=16
  state state_magic_number_0
    OutputState=0
  state state_magic_number_01
    OutputState=1
  state state_magic_number_02
    OutputState=2
  state state_magic_number_03
    OutputState=3
  state state_timestamp_0
    OutputState=4
  state state_timestamp_01
    OutputState=5
  state state_DC_sample
    OutputState=6
    count_chs=count_chs+1
  state state_chan_sample
    OutputState=7
  state state_stim_on_off
    OutputState=8
    count_chs=0
    count_stim_on_off=count_stim_on_off+1
  state state_stim_pol
    OutputState=9
    count_stim_on_off=0
    count_stim_pol=count_stim_pol+1
  state state_amp_settle
    OutputState=10
    count_stim_pol=0
    count_amp_settle=count_amp_settle+1
  state state_charge_recov
    OutputState=11
    count_amp_settle=0
    count_state_charge=count_state_charge+1
  state state_DAC
    OutputState=12
    count_state_charge=0
    count_1=count_1+1
  state state_ADC
    OutputState=13
    count_1=0
    count_2=count_2+1
  state state_TTL_in
    count_2=0
    OutputState=14
  state state_TTL_out
    OutputState=15
  (default) -> idle_state
  state_TTL_out -> idle_state
  idle_state -> state_magic_number_0 : [input_state==8]
  state_magic_number_0 -> state_magic_number_01
  state_magic_number_01 -> state_magic_number_02
  state_magic_number_02 -> state_magic_number_03
  state_magic_number_03 -> state_timestamp_0
  state_timestamp_0 -> state_timestamp_01
  state_timestamp_01 -> state_DC_sample
  state_chan_sample -> state_DC_sample [order 1] : [count_chs<160]
  state_DC_sample -> state_chan_sample
  state_chan_sample -> state_stim_on_off [order 2] : [count_chs==160]
  state_stim_on_off -> state_stim_pol : [count_stim_on_off==8]
  state_stim_pol -> state_amp_settle : [count_stim_pol==8]
  state_amp_settle -> state_charge_recov : [count_amp_settle==8]
  state_charge_recov -> state_DAC : [count_state_charge==8]
  state_DAC -> state_DAC [order 2]
  state_DAC -> state_ADC [order 1] : [count_1==8]
  state_ADC -> state_ADC [order 2]
  state_ADC -> state_TTL_in [order 1] : [count_2==8]
  state_TTL_in -> state_TTL_out
  data: OutputState output uint8 =uint8(0); count_1 local uint8 =uint8(0); count_2 local uint8 =uint8(0); input_state input uint8; count_stim_pol local uint8 =uint8(0); count_stim_on_off local uint8 =uint8(0); count_amp_settle local uint8 =uint8(0); count_state_charge local uint8 =uint8(0); count_chs local uint8 =uint8(0)

== stateflow chart gm_CustArch_vnl/cust_architecture_vnl/input_interpret_store_retrieve/InputStateMachine ==
  settings: sampleTime=1/1e6  stateMachineType=MOORE_MACHINE  initializeOutput=1
  state state_magic_number_0
    InputState=0
  state state_magic_number_01
    InputState=1
  state state_magic_number_02
    InputState=2
  state state_magic_number_03
    InputState=3
  state state_timestamp_0
    InputState=4
  state state_timestamp_01
    InputState=5
  state state_DC_sample
    InputState=6
  state state_chan_sample
    InputState=7
  state state_stim_on_off
    InputState=8
  state state_stim_pol
    InputState=9
  state state_amp_settle
    InputState=10
  state state_charge_recov
    InputState=11
  state state_DAC1
    InputState=12
    count_1=count_1
  state state_DAC
    InputState=12
    count_1=count_1+1
  note: Bad state machine?
      | Probably I should use converter counter but it works
      | so let's keep like this for now
  state state_ADC
    InputState=13
    count_1=0
    count_2=count_2+1
  state state_ADC1
    InputState=13
    count_1=0
    count_2=count_2
  state state_TTL_in
    count_2=0
    InputState=14
  state state_TTL_out
    InputState=15
  (default) -> state_magic_number_0
  state_TTL_out -> state_magic_number_0
  state_magic_number_03 -> state_magic_number_0 [order 2]
  state_timestamp_0 -> state_magic_number_0 [order 2]
  state_magic_number_02 -> state_magic_number_0 [order 2]
  state_magic_number_01 -> state_magic_number_0 [order 2]
  state_magic_number_0 -> state_magic_number_01 : [FIFO_data_in==12043 &  FIFO_write_to==1]
  state_magic_number_01 -> state_magic_number_02 [order 1] : [FIFO_data_in==18801 &  FIFO_write_to==1]
  state_magic_number_02 -> state_magic_number_03 [order 1] : [FIFO_data_in==11402 &  FIFO_write_to==1]
  state_magic_number_03 -> state_timestamp_0 [order 1] : [FIFO_data_in==36180 &  FIFO_write_to==1]
  state_timestamp_0 -> state_timestamp_01 [order 1] : [FIFO_write_to==1]
  state_timestamp_01 -> state_DC_sample : [FIFO_write_to==1]
  state_chan_sample -> state_DC_sample [order 1] : [channel_0_19<20 & FIFO_write_to==1]
  state_DC_sample -> state_stim_on_off [order 2] : [channel_0_19==20 ]
  state_DC_sample -> state_chan_sample [order 1] : [FIFO_write_to==1 & channel_0_19<20]
  state_chan_sample -> state_stim_on_off [order 2] : [channel_0_19==20 & inc_source_device_MSB==1 & FIFO_write_to==1]
  state_stim_on_off -> state_stim_pol : [inc_source_device_MSB==1]
  state_stim_pol -> state_amp_settle : [inc_source_device_MSB==1]
  state_amp_settle -> state_charge_recov : [ inc_source_device_MSB==1]
  state_charge_recov -> state_DAC : [inc_source_device_MSB==1]
  state_DAC -> state_DAC1 [order 3] : [FIFO_write_to==0]
  state_DAC -> state_DAC [order 2] : [FIFO_write_to==1]
  state_DAC1 -> state_DAC : [FIFO_write_to==1]
  state_DAC -> state_ADC [order 1] : [count_1==8]
  state_ADC -> state_ADC1 [order 3] : [FIFO_write_to==0]
  state_ADC -> state_ADC [order 2] : [FIFO_write_to==1]
  state_ADC1 -> state_ADC : [FIFO_write_to==1]
  state_ADC -> state_TTL_in [order 1] : [count_2==8]
  state_TTL_in -> state_TTL_out : [FIFO_write_to==1]
  data: FIFO_data_in input; FIFO_write_to input; InputState output uint8; channel_0_19 input; count_1 local uint8 [0..8] =uint8(0); count_2 local uint8 [0..8] =uint8(0); inc_source_device_MSB input

== stateflow chart gm_CustArch_vnl/cust_architecture/input_interpret_store_retrieve/InputStateMachine/InputStateMachine ==
  settings: sampleTime=1/1e6  stateMachineType=MOORE_MACHINE  initializeOutput=1
  state state_magic_number_0
    InputState=0
  state state_magic_number_01
    InputState=1
  state state_magic_number_02
    InputState=2
  state state_magic_number_03
    InputState=3
  state state_timestamp_0
    InputState=4
  state state_timestamp_01
    InputState=5
  state state_DC_sample
    InputState=6
  state state_chan_sample
    InputState=7
  state state_stim_on_off
    InputState=8
  state state_stim_pol
    InputState=9
  state state_amp_settle
    InputState=10
  state state_charge_recov
    InputState=11
  state state_DAC1
    InputState=12
    count_1=count_1
  state state_DAC
    InputState=12
    count_1=count_1+1
  note: Bad state machine?
      | Probably I should use converter counter but it works
      | so let's keep like this for now
  state state_ADC
    InputState=13
    count_1=0
    count_2=count_2+1
  state state_ADC1
    InputState=13
    count_1=0
    count_2=count_2
  state state_TTL_in
    count_2=0
    InputState=14
  state state_TTL_out
    InputState=15
  (default) -> state_magic_number_0
  state_TTL_out -> state_magic_number_0
  state_magic_number_03 -> state_magic_number_0 [order 2]
  state_timestamp_0 -> state_magic_number_0 [order 2]
  state_magic_number_02 -> state_magic_number_0 [order 2]
  state_magic_number_01 -> state_magic_number_0 [order 2]
  state_magic_number_0 -> state_magic_number_01 : [FIFO_data_in==12043 &  FIFO_write_to==1]
  state_magic_number_01 -> state_magic_number_02 [order 1] : [FIFO_data_in==18801 &  FIFO_write_to==1]
  state_magic_number_02 -> state_magic_number_03 [order 1] : [FIFO_data_in==11402 &  FIFO_write_to==1]
  state_magic_number_03 -> state_timestamp_0 [order 1] : [FIFO_data_in==36180 &  FIFO_write_to==1]
  state_timestamp_0 -> state_timestamp_01 [order 1] : [FIFO_write_to==1]
  state_timestamp_01 -> state_DC_sample : [FIFO_write_to==1]
  state_chan_sample -> state_DC_sample [order 1] : [channel_0_19<20 & FIFO_write_to==1]
  state_DC_sample -> state_stim_on_off [order 2] : [channel_0_19==20 ]
  state_DC_sample -> state_chan_sample [order 1] : [FIFO_write_to==1 & channel_0_19<20]
  state_chan_sample -> state_stim_on_off [order 2] : [channel_0_19==20 & inc_source_device_MSB==1 & FIFO_write_to==1]
  state_stim_on_off -> state_stim_pol : [inc_source_device_MSB==1]
  state_stim_pol -> state_amp_settle : [inc_source_device_MSB==1]
  state_amp_settle -> state_charge_recov : [ inc_source_device_MSB==1]
  state_charge_recov -> state_DAC : [inc_source_device_MSB==1]
  state_DAC -> state_DAC1 [order 3] : [FIFO_write_to==0]
  state_DAC -> state_DAC [order 2] : [FIFO_write_to==1]
  state_DAC1 -> state_DAC : [FIFO_write_to==1]
  state_DAC -> state_ADC [order 1] : [count_1==8]
  state_ADC -> state_ADC1 [order 3] : [FIFO_write_to==0]
  state_ADC -> state_ADC [order 2] : [FIFO_write_to==1]
  state_ADC1 -> state_ADC : [FIFO_write_to==1]
  state_ADC -> state_TTL_in [order 1] : [count_2==8]
  state_TTL_in -> state_TTL_out : [FIFO_write_to==1]
  data: FIFO_data_in input; FIFO_write_to input; InputState output uint8; channel_0_19 input; count_1 local uint8 [0..8] =uint8(0); count_2 local uint8 [0..8] =uint8(0); inc_source_device_MSB input

== stateflow chart gm_CustArch_vnl/cust_architecture_vnl/output_interpret/OutputStateMachine ==
  settings: sampleTime=1/1e6  stateMachineType=MOORE_MACHINE  initializeOutput=1
  state idle_state
    OutputState=16
  state state_magic_number_0
    OutputState=0
  state state_magic_number_01
    OutputState=1
  state state_magic_number_02
    OutputState=2
  state state_magic_number_03
    OutputState=3
  state state_timestamp_0
    OutputState=4
  state state_timestamp_01
    OutputState=5
  state state_DC_sample
    OutputState=6
    count_chs=count_chs+1
  state state_chan_sample
    OutputState=7
  state state_stim_on_off
    OutputState=8
    count_chs=0
    count_stim_on_off=count_stim_on_off+1
  state state_stim_pol
    OutputState=9
    count_stim_on_off=0
    count_stim_pol=count_stim_pol+1
  state state_amp_settle
    OutputState=10
    count_stim_pol=0
    count_amp_settle=count_amp_settle+1
  state state_charge_recov
    OutputState=11
    count_amp_settle=0
    count_state_charge=count_state_charge+1
  state state_DAC
    OutputState=12
    count_state_charge=0
    count_1=count_1+1
  state state_ADC
    OutputState=13
    count_1=0
    count_2=count_2+1
  state state_TTL_in
    count_2=0
    OutputState=14
  state state_TTL_out
    OutputState=15
  (default) -> idle_state
  state_TTL_out -> idle_state
  idle_state -> state_magic_number_0 : [input_state==8]
  state_magic_number_0 -> state_magic_number_01
  state_magic_number_01 -> state_magic_number_02
  state_magic_number_02 -> state_magic_number_03
  state_magic_number_03 -> state_timestamp_0
  state_timestamp_0 -> state_timestamp_01
  state_timestamp_01 -> state_DC_sample
  state_chan_sample -> state_DC_sample [order 1] : [count_chs<160]
  state_DC_sample -> state_chan_sample
  state_chan_sample -> state_stim_on_off [order 2] : [count_chs==160]
  state_stim_on_off -> state_stim_pol : [count_stim_on_off==8]
  state_stim_pol -> state_amp_settle : [count_stim_pol==8]
  state_amp_settle -> state_charge_recov : [count_amp_settle==8]
  state_charge_recov -> state_DAC : [count_state_charge==8]
  state_DAC -> state_DAC [order 2]
  state_DAC -> state_ADC [order 1] : [count_1==8]
  state_ADC -> state_ADC [order 2]
  state_ADC -> state_TTL_in [order 1] : [count_2==8]
  state_TTL_in -> state_TTL_out
  data: OutputState output uint8 =uint8(0); count_1 local uint8 =uint8(0); count_2 local uint8 =uint8(0); input_state input uint8; count_stim_pol local uint8 =uint8(0); count_stim_on_off local uint8 =uint8(0); count_amp_settle local uint8 =uint8(0); count_state_charge local uint8 =uint8(0); count_chs local uint8 =uint8(0)
